simulink model "EnergyCommunity"  (R2022b)
settings: Solver=VariableStepAuto  StartTime=0.0  StopTime=5  RelTol=1e-3
(part 2 of 2)

== matlab function EnergyCommunity/media2 ==
  data: u input; y output
function y = media(u)

y = mean(u);
